simulink model "Assgn_2_18EE35014_Part_1"  (R2020b)
settings: Solver=VariableStepAuto  StartTime=0.0  StopTime=1000  RelTol=1e-9
settings Model: Creator=Pratyush Jaiswal  LastModifiedBy=Pratyush Jaiswal

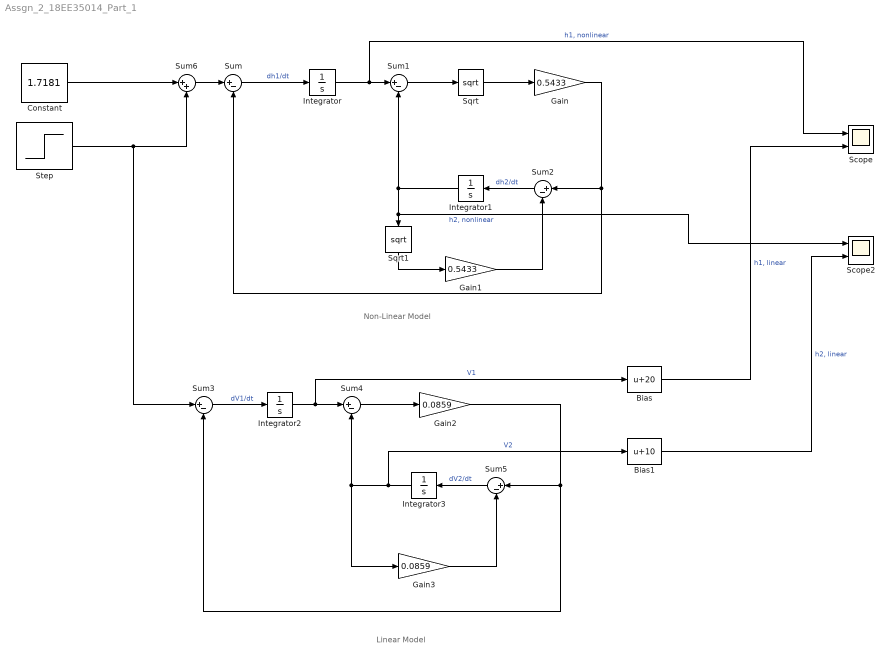
== system Assgn_2_18EE35014_Part_1 ==
  note: Non-Linear Model
  note: Linear Model
  Bias : Bias  Bias=20
  Bias1 : Bias  Bias=10
  Constant : Constant  Value=1.7181
  Gain : Gain  Gain=0.5433
  Gain1 : Gain  Gain=0.5433
  Gain2 : Gain  Gain=0.0859
  Gain3 : Gain  Gain=0.0859
  Integrator{,1..3} (4 alike) : Integrator
  Scope : Scope  NumInputPorts=2
  Scope2 : Scope  NumInputPorts=2
  Sqrt : Sqrt  SaturateOnIntegerOverflow=on
  Sqrt1 : Sqrt  SaturateOnIntegerOverflow=on
  Step : Step  Time=500  After=0.0625  SampleTime=0
  Sum{,1..5} (6 alike) : Sum  Inputs=|+-
  Sum6 : Sum  Inputs=|++
  wires:
  Constant/1 -> Sum6/1
  Sum/1 -> Integrator/1  "dh1/dt"
  Integrator/1 -> Scope/1, Sum1/1  "h1, nonlinear"
  Sum1/1 -> Sqrt/1
  Sqrt/1 -> Gain/1
  Gain/1 -> Sum/2, Sum2/1
  Sum2/1 -> Integrator1/1  "dh2/dt"
  Integrator1/1 -> Scope2/1, Sqrt1/1, Sum1/2  "h2, nonlinear"
  Sqrt1/1 -> Gain1/1
  Gain1/1 -> Sum2/2
  Sum3/1 -> Integrator2/1  "dV1/dt"
  Integrator2/1 -> Bias/1, Sum4/1  "V1"
  Sum4/1 -> Gain2/1
  Gain3/1 -> Sum5/2
  Integrator3/1 -> Bias1/1, Sum4/2, Gain3/1  "V2"
  Sum5/1 -> Integrator3/1  "dV2/dt"
  Gain2/1 -> Sum5/1, Sum3/2
  Bias1/1 -> Scope2/2  "h2, linear"
  Sum6/1 -> Sum/1
  Step/1 -> Sum3/1, Sum6/2
  Bias/1 -> Scope/2  "h1, linear"
